simulink model "INTER_IIT_3rdorder_without_noise_DSM"  (R2024a)
settings: Solver=VariableStepAuto  StartTime=0.0  StopTime=1000000  RelTol=1e-3
undefined symbols (not defined in the file): DiscIntNeverNeededParam
settings Model: Creator=Siddhant  LastModifiedBy=somya

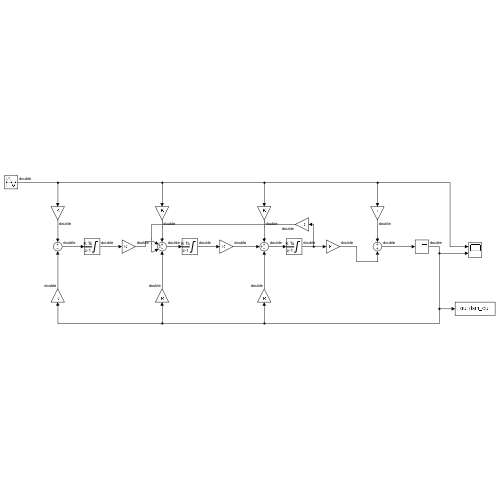
[thumbnail: Simulink's stored preview of the top-level diagram]
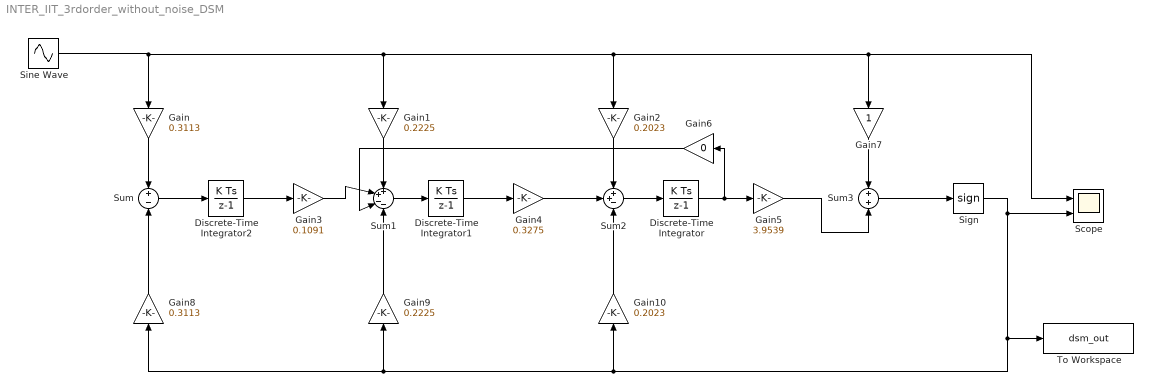
== system INTER_IIT_3rdorder_without_noise_DSM ==
  Discrete-Time Integrator : DiscreteIntegrator  gainval=1  SampleTime=0.1  LimitOutput=on  UpperSaturationLimit=1.8  LowerSaturationLimit=-1.8  ICPrevOutput=DiscIntNeverNeededParam  ICPrevScaledInput=DiscIntNeverNeededParam
  Discrete-Time Integrator1 : DiscreteIntegrator  gainval=1  SampleTime=0.1  LimitOutput=on  UpperSaturationLimit=1.8  LowerSaturationLimit=-1.8  ICPrevOutput=DiscIntNeverNeededParam  ICPrevScaledInput=DiscIntNeverNeededParam
  Discrete-Time Integrator2 : DiscreteIntegrator  gainval=1  SampleTime=0.1  LimitOutput=on  UpperSaturationLimit=1.8  LowerSaturationLimit=-1.8  ICPrevOutput=DiscIntNeverNeededParam  ICPrevScaledInput=DiscIntNeverNeededParam
  Gain : Gain  Gain=0.3113
  Gain1 : Gain  Gain=0.2225
  Gain10 : Gain  Gain=0.2023
  Gain2 : Gain  Gain=0.2023
  Gain3 : Gain  Gain=0.1091
  Gain4 : Gain  Gain=0.3275
  Gain5 : Gain  Gain=3.9539
  Gain6 : Gain  Gain=0
  Gain7 : Gain
  Gain8 : Gain  Gain=0.3113
  Gain9 : Gain  Gain=0.2225
  Scope : Scope  NumInputPorts=2
  Sign : Signum
  Sine Wave : Sin  SineType=Sample based  Amplitude=0.5  Frequency=500*2*3.14  Samples=8192000  SampleTime=0.1
  Sum : Sum  Inputs=+-
  Sum1 : Sum  Inputs=++--
  Sum2 : Sum  Inputs=++-
  Sum3 : Sum
  To Workspace : ToWorkspace  VariableName=dsm_out  SampleTime=-1
  wires:
  Sum2/1 -> Discrete-Time Integrator/1
  Discrete-Time Integrator/1 -> Gain6/1, Gain5/1
  Sum1/1 -> Discrete-Time Integrator1/1
  Discrete-Time Integrator1/1 -> Gain4/1
  Gain6/1 -> Sum1/3
  Gain8/1 -> Sum/2
  Gain4/1 -> Sum2/2
  Gain10/1 -> Sum2/3
  Gain/1 -> Sum/1
  Sum/1 -> Discrete-Time Integrator2/1
  Gain2/1 -> Sum2/1
  Gain1/1 -> Sum1/1
  Gain3/1 -> Sum1/2
  Gain7/1 -> Sum3/1
  Gain5/1 -> Sum3/2
  Gain9/1 -> Sum1/4
  Discrete-Time Integrator2/1 -> Gain3/1
  Sum3/1 -> Sign/1
  Sign/1 -> To Workspace/1, Gain10/1, Gain9/1, Gain8/1, Scope/2
  Sine Wave/1 -> Gain2/1, Scope/1, Gain7/1, Gain1/1, Gain/1
